simulink model "TurtleBot"  (R2023b)
settings: Solver=VariableStepAuto  StartTime=0.0  StopTime=90  RelTol=1e-3
settings Model: Creator=lerio  LastModifiedBy=lerio

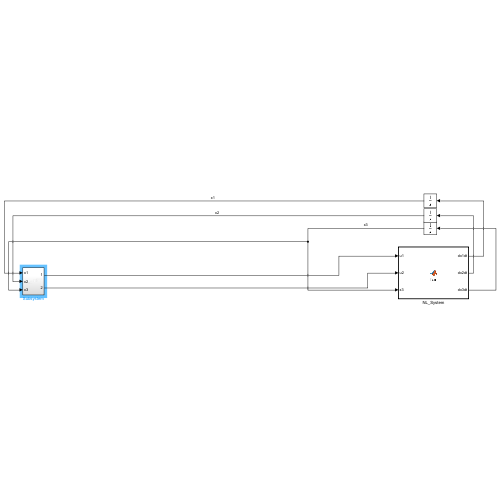
[thumbnail: Simulink's stored preview of the top-level diagram]
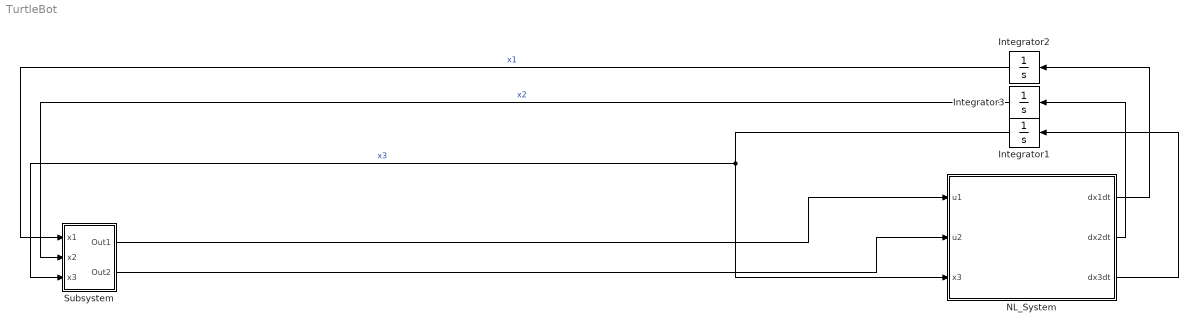
== system TurtleBot ==
  Integrator1 : Integrator  InitialCondition=0.1
  Integrator2 : Integrator  InitialCondition=0.1
  Integrator3 : Integrator
  NL_System : MATLAB Function  TreatAsAtomicUnit=on
  Subsystem : Subsystem
  wires:
  NL_System/3(dx3dt) -> Integrator1/1
  Integrator1/1 -> Subsystem/3(x3), NL_System/3(x3)  "x3"
  NL_System/1(dx1dt) -> Integrator2/1
  NL_System/2(dx2dt) -> Integrator3/1
  Integrator2/1 -> Subsystem/1(x1)  "x1"
  Integrator3/1 -> Subsystem/2(x2)  "x2"
  Subsystem/1(Out1) -> NL_System/1(u1)
  Subsystem/2(Out2) -> NL_System/2(u2)

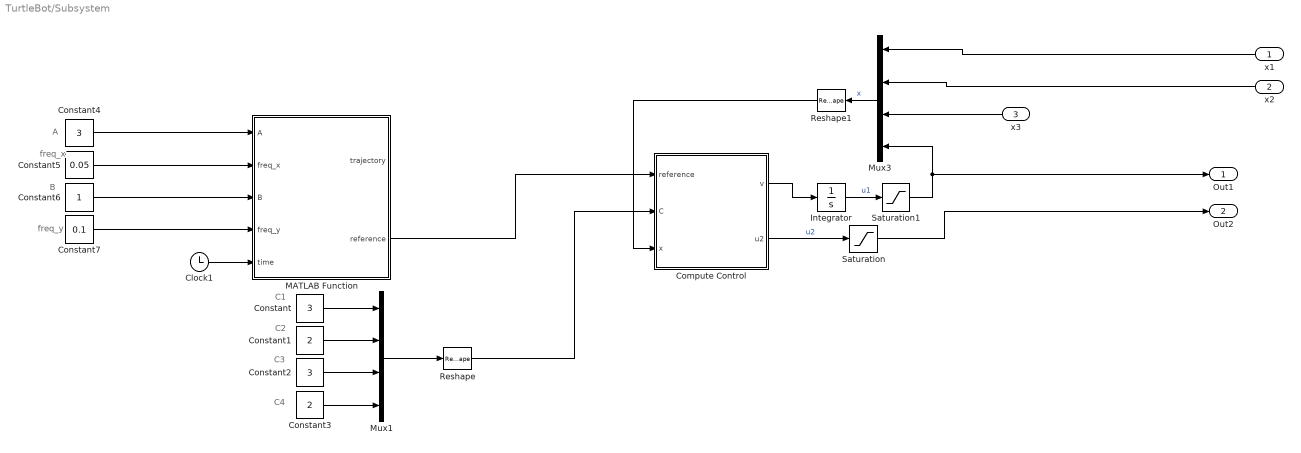
== system TurtleBot/Subsystem ==
  note: freq_y
  note: B
  note: freq_x
  note: A
  note: C2
  note: C1
  note: C4
  note: C3
  x1 : Inport
  x2 : Inport  Port=2
  x3 : Inport  Port=3
  Clock1 : Clock
  Compute Control : MATLAB Function  TreatAsAtomicUnit=on
  Constant : Constant  Value=3  SampleTime=-1
  Constant1 : Constant  Value=2  SampleTime=-1
  Constant2 : Constant  Value=3  SampleTime=-1
  Constant3 : Constant  Value=2  SampleTime=-1
  Constant4 : Constant  Value=3  SampleTime=-1
  Constant5 : Constant  Value=0.05  SampleTime=-1
  Constant6 : Constant  SampleTime=-1
  Constant7 : Constant  Value=0.1  SampleTime=-1
  Integrator : Integrator  InitialCondition=0.1
  MATLAB Function : MATLAB Function  TreatAsAtomicUnit=on
  Mux1 : Mux
  Mux3 : Mux
  Reshape : Reshape  OutputDimensionality=Column vector (2-D)
  Reshape1 : Reshape  OutputDimensionality=Column vector (2-D)
  Saturation : Saturate  UpperLimit=0.8  LowerLimit=-0.8
  Saturation1 : Saturate  UpperLimit=0.15  LowerLimit=-0.15
  Out1 : Outport
  Out2 : Outport  Port=2
  wires:
  Constant2/1 -> Mux1/3
  Mux1/1 -> Reshape/1
  Saturation1/1 -> Out1/1, Mux3/4
  x1/1 -> Mux3/1
  Saturation/1 -> Out2/1
  Constant1/1 -> Mux1/2
  Constant3/1 -> Mux1/4
  Constant7/1 -> MATLAB Function/4(freq_y)
  x2/1 -> Mux3/2
  Constant6/1 -> MATLAB Function/3(B)
  Constant/1 -> Mux1/1
  Reshape1/1 -> Compute Control/3(x)
  Compute Control/1(v) -> Integrator/1
  Constant4/1 -> MATLAB Function/1(A)
  Compute Control/2(u2) -> Saturation/1  "u2"
  Constant5/1 -> MATLAB Function/2(freq_x)
  MATLAB Function/2(reference) -> Compute Control/1(reference)
  Reshape/1 -> Compute Control/2(C)
  Clock1/1 -> MATLAB Function/5(time)
  Integrator/1 -> Saturation1/1  "u1"
  Mux3/1 -> Reshape1/1  "x"
  x3/1 -> Mux3/3

== matlab function TurtleBot/NL_System ==
  data: u1 input; u2 input; dx1dt output; dx2dt output; dx3dt output; x3 input
function [dx1dt, dx2dt, dx3dt] = fcn(u1,u2, x3)

dx1dt = cos(x3)*u1;
dx2dt = sin(x3)*u1;
dx3dt = u2;

== matlab function TurtleBot/Subsystem/Compute Control ==
  data: reference input; v output; C input; x input; u2 output
function [v,u2] = fcn(reference, C, x)

Bc = [ cos(x(3)), -sin(x(3))*x(4);
       sin(x(3)),  cos(x(3))*x(4)];

M1 = [reference(3);
      reference(6)];

M2 = [C(1)*(x(1) - reference(1)) + C(2)*(cos(x(3))*x(4) - reference(2));
      C(3)*(x(2) - reference(4)) + C(4)*(sin(x(3))*x(4) - reference(5))];

U = Bc\(M1-M2);

v = U(1);
u2 = U(2);

== matlab function TurtleBot/Subsystem/MATLAB Function ==
  data: trajectory output; reference output; A input; freq_x input; B input; freq_y input; time input
function [trajectory,reference] = fcn(A, freq_x, B, freq_y, time)

Xdes = A * sin(freq_x * time);
Ydes = B * sin(freq_y * time);

Xdes_dot = A * freq_x * cos(freq_x * time);
Ydes_dot = B * freq_y * cos(freq_y * time);

Xdes_2dot = - A * freq_x^2 * sin(freq_x * time);
Ydes_2dot = - B * freq_y^2 * sin(freq_y * time);

reference = [Xdes;
            Xdes_dot;
            Xdes_2dot;
            Ydes;
            Ydes_dot;
            Ydes_2dot];

trajectory = [Xdes;
              Ydes];
